simulink model "motor_ctrl_dtc_ver1"  (R2020b)
settings: Solver=VariableStepAuto  StartTime=0.0  StopTime=1  RelTol=1e-3
InitFcn:
  | Rs=0.43;
  | 
  | Lls=0.002
  | 
  | Rr=0.816;
  | 
  | Llr=0.002
  | 
  | Lm=0.6931;
  | 
  | 
  | J=0.085;
  | np=2;
  | 
  | Ts=1e-5;
  | 
  | Udc=400*sqrt(3)
  | Tpwm = 1e-4;
  | 
  | 
  | 
  | Ls = 1.5*Lm+Lls
  | Lr = 1.5*Lm+Llr
  | Tr = Lr/Rr;
  | sigma = (Ls*Lr-Lm*Lm)/Ls/Lr;
model workspace (MAT data in the model file):
  Tsys = 2e-06
  sample_time = 1e-06
libraries: powerlib x17, simulink x3
settings Model: SimulationMode=accelerator  OrderedModelArguments=off  Creator=messer  LastModifiedBy=messer

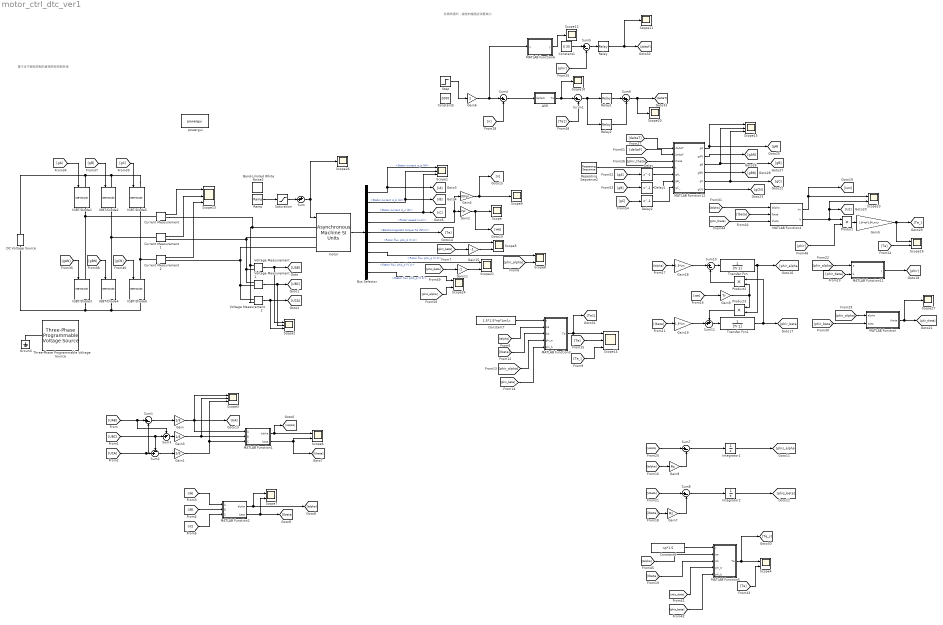
== system motor_ctrl_dtc_ver1 ==
  note: 在高转速时，磁链的幅值应该要减小
  note: 基于定子磁链控制的直接转矩控制系统
  ASR : Subsystem
  Band-Limited White Noise2 : simulink/Sources/Band-Limited White Noise  Cov=[0.0001]  Ts=1e-4  seed=[130341]
  Bus Selector : BusSelector  OutputSignals=Stator measurements.Stator current is_a (A),Stator measurements.Stator current is_b (A),Stator measurements.Stator current is_c (A),Mechanical.Rotor speed (wm),Mechanical.Electromagnetic torque Te (N*m),Rotor measurements.Rotor flux phir_d (V s),Rotor measurements.Rotor flux phir_q (V s),Stator measurements.Stator flux phis_d (V s),Stator measurements.Stator flux phis_q (V s)
  Constant1 : Constant  Value=0.35
  Constant5 : Constant  Value=2000
  Constant6 : Constant  Value=np*1.5
  Constant7 : Constant  Value=1.5*1.5*np*Lm/Lr
  Current Measurement : powerlib/Measurements/Current Measurement  PhasorSimulation=off  OutputType=Complex  PSBequivalent=0
  Current Measurement1 : powerlib/Measurements/Current Measurement  PhasorSimulation=off  OutputType=Complex  PSBequivalent=0
  Current Measurement2 : powerlib/Measurements/Current Measurement  PhasorSimulation=off  OutputType=Complex  PSBequivalent=0
  DC Voltage Source : powerlib/Electrical Sources/DC Voltage Source  Amplitude=Udc  Measurements=None
  Delay : Delay  DelayLength=1  InitialCondition=0
  Delay1 : Delay  DelayLength=1  InitialCondition=0
  Delay2 : Delay  DelayLength=1  InitialCondition=0
  Gain : Gain  Gain=1/3
  Gain1 : Gain  Gain=1/3
  Gain11 : Gain  Gain=-1
  Gain15 : Gain  Gain=-1
  Gain18 : Gain  Gain=1.5*Lm
  Gain19 : Gain  Gain=1.5*Lm
  Gain2 : Gain  Gain=np
  Gain3 : Gain  Gain=1/3
  Gain4 : Gain  Gain=30/pi
  Gain5 : Gain  Gain=1.5*np*1.5*Lm/Lr
  Gain6 : Gain
  Gain7 : Gain  Gain=Rs
  Gain8 : Gain  Gain=Rs
  Gain9 : Gain  Gain=Tr
  Ground : powerlib/Elements/Ground  LConnTagsString=a
  IGBT/Diode{1..6} (6 alike) : powerlib/Power Electronics/IGBT//Diode  Ron=1e-3  Rs=1e5  Cs=inf  Measurements=on
  Integrator1 : Integrator
  Integrator2 : Integrator
  MATLAB Function : MATLAB Function  TreatAsAtomicUnit=on
  MATLAB Function1 : MATLAB Function  TreatAsAtomicUnit=on
  MATLAB Function11 : MATLAB Function  TreatAsAtomicUnit=on
  MATLAB Function12 : MATLAB Function  TreatAsAtomicUnit=on
  MATLAB Function2 : MATLAB Function  TreatAsAtomicUnit=on
  MATLAB Function3 : MATLAB Function  TreatAsAtomicUnit=on
  MATLAB Function4 : MATLAB Function  TreatAsAtomicUnit=on
  MATLAB Function5 : MATLAB Function  TreatAsAtomicUnit=on
  MATLAB Function6 : MATLAB Function  TreatAsAtomicUnit=on
  Product : Product
  Product2 : Product
  Product3 : Product
  Ramp : simulink/Sources/Ramp  slope=100  start=0.25  InitialOutput=5
  Relay : Relay  OnSwitchValue=0.1  OffSwitchValue=-0.1
  Relay1 : Relay  OnSwitchValue=15  OffSwitchValue=10
  Relay2 : Relay  OnSwitchValue=-10  OffSwitchValue=-15  OnOutputValue=0  OffOutputValue=-1
  Repeating Sequence2 : simulink/Sources/Repeating Sequence  rep_seq_t=[0 Tpwm]  rep_seq_y=[0 1]
  Saturation : Saturate  UpperLimit=20  LowerLimit=0
  Scope{,9..12,20,26..27} (8 alike) : Scope
  Scope{1..3,13..15} (6 alike) : Scope  NumInputPorts=3
  Scope{4..8,16,21,23..24} (9 alike) : Scope  NumInputPorts=2
  Step : Step  Time=0.21  Before=2000  After=3000  SampleTime=0
  Su`m1 : Sum  Inputs=|+-
  Sum : Sum  Inputs=++|
  Sum{1,4..5,7..8,10} (6 alike) : Sum  Inputs=|+-
  Sum11 : Sum  Inputs=++|
  Sum2 : Sum  Inputs=-+|
  Sum3 : Sum  Inputs=-+|
  Sum6 : Sum  Inputs=|++
  Three-Phase Programmable Voltage Source : powerlib/Electrical Sources/Three-Phase Programmable Voltage Source  PositiveSequence="[380/sqrt(2)  0 50]"  VariationEntity=None  VariationType=Table of time-amplitude pairs  VariationTypeAlt=Step  VariationStep=0.5  VariationRate=10  VariationMagnitude=0.3  VariationFrequency=2  VariationTiming=[1 2]  VariationPhaseA=off  Amplitudes=[1 0.8 1.2 1.0]  TimeValues=[0 0.1 0.15 0.2]  HarmonicGeneration=off  HarmonicA=[3 0.2 -25 0]  HarmonicB=[2 0.15 35 2]  Timing="[0.05  3]"  BusType=swing  Pref=0  Qref=0  Qmin=-inf  Qmax=inf
  Transfer Fcn : TransferFcn  Denominator=[Tr 1]
  Transfer Fcn1 : TransferFcn  Denominator=[Tr 1]
  Voltage Measurement : powerlib/Measurements/Voltage Measurement  PhasorSimulation=off  OutputType=Complex  PSBequivalent=0
  Voltage Measurement1 : powerlib/Measurements/Voltage Measurement  PhasorSimulation=off  OutputType=Complex  PSBequivalent=0
  Voltage Measurement2 : powerlib/Measurements/Voltage Measurement  PhasorSimulation=off  OutputType=Complex  PSBequivalent=0
  motor : powerlib/Machines/Asynchronous Machine SI Units  RotorType=Squirrel-cage  PresetModel=No  MechanicalLoad=Torque Tm  ShowDetailedParameters=on  ReferenceFrame=Stationary  Units=SI  MeasurementBus=off  NominalParameters=[562000 2750 135]  Stator=[Rs Lls]  Rotor=[Rr Llr]  Cage1=[0.4155 0.002066]  Cage2=[0.4168 0.0003495]  Lm=Lm  Mechanical=[J 0 np]  PolePairs=2  InitialConditions=[1 0 0 0 0 0 0 0]  SimulateSaturation=off  Saturation=[14.03593122, 27.81365428, 53.79336849, 72.68890987, 97.98006896, 148.6815601, 215.7428561, 302.9841135, 428.7778367 ; 230, 322, 414, 460, 506, 552, 598, 644, 690]  LoadFlowParameters=1492000  TsPowergui=0  TsBlock=-1  IterativeModel=Trapezoidal non iterative  IterativeDiscreteModel=Trapezoidal non iterative  Pmec=1.492e+006
  powergui : powerlib/powergui  Priority=1  SimulationMode=Discrete  SampleTime=Tsys  frequency=60  Iterations=50  frequencyindice=0  Pbase=100e6  ErrMax=1e-4  UnitsV=kV  UnitsW=MW  buscounter=0  FunctionMessages=off  echomessages=off  EnableUseOfTLC=off  CurrentSourceSwitches=off  DisableSnubberDevices=off  DisableRonSwitches=off  DisableVfSwitches=off  DisplayEquations=off  AutomaticDiscreteSolvers=off  SolverType=Tustin/Backward Euler (TBE)  Interpol=off  ExternalGateDelay=off  methode=off  Ts=100  x0status=blocks  SPID=on  SwTol=0  HookPort=off  NonlinearTolerance=1e-4  nMaxIteration=100  ContinueOnMaxIteration=off  RestoreLinks=warning  ResistiveCurrentMeasurement=off  Frange=[0:2:500]  Ylog=off  Xlog=on  ShowGrid=off  save=off  variable=ZData  structure=0  ZoomFFT=off  StartTime=0.0  cycles=1  DisplayStyle=1  fundamental=60  FreqAxis=off  MaxFrequency=1000  frequencyindicesteady=1  RmsSteady=1  display=off
  wires:
  Bus Selector/4 -> Gain4/1, Gain2/1  "<Rotor speed (wm)>"
  Bus Selector/2 -> [iB], Scope1/2  "<Stator current is_b (A)>"
  Bus Selector/5 -> [Te]  "<Electromagnetic torque Te (N*m)>"
  Saturation/1 -> Sum/2
  Bus Selector/1 -> [iA], Scope1/1  "<Stator current is_a (A)>"
  motor/1 -> Bus Selector/1
  Bus Selector/3 -> [iC], Scope1/3  "<Stator current is_c (A)>"
  Ramp/1 -> Saturation/1
  Voltage Measurement1/1 -> [UBC], Scope2/2
  Voltage Measurement/1 -> Scope2/1, [UAB]
  Voltage Measurement2/1 -> [UCA], Scope2/3
  [UAB] -> Sum3/1, Sum1/1
  [UCA] -> Sum1/2, Sum2/2
  Sum1/1 -> Gain/1
  [UBC] -> Sum2/1, Sum3/2
  Sum2/1 -> Gain1/1
  Sum3/1 -> Gain3/1
  Gain3/1 -> MATLAB Function1/2(B), Scope3/2
  Gain/1 -> MATLAB Function1/1(A), [UA], Scope3/1
  Gain1/1 -> MATLAB Function1/3(C), Scope3/3
  Sum/1 -> Scope26/1, motor/1
  MATLAB Function1/1(alpha) -> [Ualpha], Scope6/1
  MATLAB Function1/2(beta) -> [Ubeta], Scope6/2
  MATLAB Function2/2(beta) -> [Ibeta], Scope7/2
  [iB] -> MATLAB Function2/2(B)
  MATLAB Function2/1(alpha) -> Scope7/1, [Ialpha]
  [phir_alpha] -> Scope8/2
  [phir_beta] -> Gain15/1
  Gain15/1 -> Scope5/2
  Bus Selector/6 -> Scope5/1  "<Rotor flux phir_d (V s)>"
  Bus Selector/7 -> Scope8/1  "<Rotor flux phir_q (V s)>"
  Gain2/1 -> [we], Scope/1
  [iA] -> MATLAB Function2/1(A)
  [iC] -> MATLAB Function2/3(C)
  Constant7/1 -> MATLAB Function3/1(c)
  [Ialpha] -> MATLAB Function3/2(isa)
  [Ibeta] -> MATLAB Function3/3(isb)
  [phir_alpha] -> MATLAB Function3/4(phi_a)
  [phir_beta] -> MATLAB Function3/5(phi_b)
  MATLAB Function3/1(Te) -> [Te1], Scope14/1
  [Te] -> Scope14/2
  Gain4/1 -> [n], Scope9/1
  Current Measurement1/1 -> Scope13/2
  Current Measurement2/1 -> Scope13/3
  Current Measurement/1 -> Scope13/1
  [Ialpha] -> MATLAB Function4/1(Ialpha)
  [Ibeta] -> MATLAB Function4/2(Ibeta)
  MATLAB Function4/2(It) -> Scope23/2, [Ist], Product/1
  Product/1 -> Gain5/1
  Gain5/1 -> [Te_], Scope16/1
  [Te] -> Scope16/2
  [phir] -> Sum5/2
  Sum5/1 -> Relay/1
  MATLAB Function4/1(Im) -> [Ism], Scope23/1
  [gA] -> IGBT/Diode1/1
  [gAN] -> IGBT/Diode3/1
  [gB] -> IGBT/Diode2/1
  [gBN] -> IGBT/Diode4/1
  [gC] -> IGBT/Diode5/1
  [gCN] -> IGBT/Diode6/1
  [phir_theta] -> MATLAB Function4/3(theta)
  [phir] -> Product/2
  [n] -> Sum4/2
  Relay/1 -> [deltaF], Scope11/1
  Sum4/1 -> ASR/1(deltaN)
  [Te1] -> Su`m1/2
  Su`m1/1 -> Relay2/1, Relay1/1
  Sum10/1 -> Transfer Fcn/1
  Gain18/1 -> Sum10/1
  Sum11/1 -> Transfer Fcn1/1
  Product2/1 -> Sum10/2
  Gain19/1 -> Sum11/2
  [Ibeta] -> Gain19/1
  [Ialpha] -> Gain18/1
  Transfer Fcn/1 -> Product3/2, [phir_alpha]
  [we] -> Gain9/1
  Product3/1 -> Sum11/1
  Gain9/1 -> Product3/1, Product2/2
  Transfer Fcn1/1 -> Product2/1, [phir_beta]
  [phir_alpha] -> MATLAB Function11/1(a)
  [phir_beta] -> MATLAB Function11/2(b)
  [phir_beta] -> MATLAB Function/2(beta)
  [phir_alpha] -> MATLAB Function/1(alpha)
  MATLAB Function11/1(y) -> [phir]
  MATLAB Function/1(theta) -> Scope27/1, [phir_theta]
  [Te_] -> Scope14/3
  ASR/1(Te) -> Su`m1/1, Scope10/1
  [phis_alpha] -> MATLAB Function5/4(phi_a)
  [Ialpha] -> MATLAB Function5/2(isa)
  [Ialpha] -> Gain8/1
  [Ibeta] -> MATLAB Function5/3(isb)
  Gain7/1 -> Sum8/2
  Integrator2/1 -> [phis_beta]
  Integrator1/1 -> [phis_alpha]
  [Te] -> Scope4/2
  [phis_beta] -> MATLAB Function5/5(phi_b)
  [Ubeta] -> Sum8/1
  Gain8/1 -> Sum7/2
  [Ibeta] -> Gain7/1
  Constant6/1 -> MATLAB Function5/1(c)
  Sum7/1 -> Integrator1/1
  MATLAB Function5/1(Te) -> Scope4/1, [Te_s]
  Sum8/1 -> Integrator2/1
  [Ualpha] -> Sum7/1
  Gain11/1 -> Scope21/2
  [phis_beta] -> Gain11/1
  Bus Selector/8 -> Scope21/1  "<Stator flux phis_d (V s)>"
  [phis_alpha] -> Scope24/2
  Bus Selector/9 -> Scope24/1  "<Stator flux phis_q (V s)>"
  Relay1/1 -> Sum6/1
  Relay2/1 -> Sum6/2
  Repeating Sequence2/1 -> MATLAB Function12/4(t)
  [phir_theta] -> MATLAB Function12/3(theta)
  Sum6/1 -> Scope20/1, [deltaT]
  [deltaT] -> MATLAB Function12/1(deltaT)
  [deltaF] -> MATLAB Function12/2(deltaF)
  MATLAB Function12/2(gAN) -> [gAN]
  MATLAB Function12/6(gCN) -> [gCN]
  MATLAB Function12/5(gC) -> Scope15/3, [gC]
  MATLAB Function12/3(gB) -> Scope15/2, [gB]
  MATLAB Function12/4(gBN) -> [gBN]
  MATLAB Function12/1(gA) -> Scope15/1, [gA]
  Delay/1 -> MATLAB Function12/5(gA_)
  [gA] -> Delay/1
  [gB] -> Delay1/1
  [gC] -> Delay2/1
  Delay1/1 -> MATLAB Function12/6(gB_)
  Delay2/1 -> MATLAB Function12/7(gC_)
  MATLAB Function6/1(y) -> Scope12/1
  Constant1/1 -> Sum5/1
  Gain6/1 -> MATLAB Function6/1(u), Sum4/1
  Step/1 -> Gain6/1
  connections:
  Voltage Measurement1/LConn1 -- Voltage Measurement/LConn2 -- motor/LConn2 -- Current Measurement1/RConn1
  Voltage Measurement2/LConn1 -- Voltage Measurement1/LConn2 -- Current Measurement2/RConn1 -- motor/LConn3
  Voltage Measurement/LConn1 -- Voltage Measurement2/LConn2 -- Current Measurement/RConn1 -- motor/LConn1
  Ground/LConn1 -- Three-Phase Programmable Voltage Source/LConn1
  IGBT/Diode2/RConn1 -- IGBT/Diode4/LConn1 -- Current Measurement1/LConn1
  IGBT/Diode5/LConn1 -- DC Voltage Source/RConn1 -- IGBT/Diode1/LConn1 -- IGBT/Diode2/LConn1
  IGBT/Diode5/RConn1 -- IGBT/Diode6/LConn1 -- Current Measurement2/LConn1
  IGBT/Diode3/RConn1 -- DC Voltage Source/LConn1 -- IGBT/Diode4/RConn1 -- IGBT/Diode6/RConn1
  IGBT/Diode1/RConn1 -- IGBT/Diode3/LConn1 -- Current Measurement/LConn1

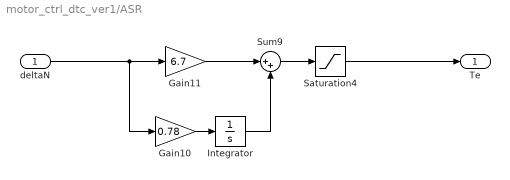
== system motor_ctrl_dtc_ver1/ASR ==
  deltaN : Inport
  Gain10 : Gain  Gain=0.78
  Gain11 : Gain  Gain=6.7
  Integrator : Integrator
  Saturation4 : Saturate  UpperLimit=300  LowerLimit=-300
  Sum9 : Sum  Inputs=|++
  Te : Outport
  wires:
  Gain11/1 -> Sum9/1
  deltaN/1 -> Gain11/1, Gain10/1
  Saturation4/1 -> Te/1
  Gain10/1 -> Integrator/1
  Sum9/1 -> Saturation4/1
  Integrator/1 -> Sum9/2

== matlab function motor_ctrl_dtc_ver1/MATLAB Function1 ==
  data: A input; alpha output; B input; C input; beta output
function [alpha, beta] = fcn(A, B, C)
k = 2/ 3;
alpha = k * (A - 0.5*B - 0.5*C);
beta = k * sqrt(3) / 2 * (B - C);

== matlab function motor_ctrl_dtc_ver1/MATLAB Function5 ==
  data: c input; Te output; isa input; isb input; phi_a input; phi_b input
function Te = fcn(c, isa, isb, phi_a, phi_b)
Te = c *( isb * phi_a - isa * phi_b);

== matlab function motor_ctrl_dtc_ver1/MATLAB Function2 ==
  data: A input; alpha output; B input; C input; beta output
function [alpha, beta] = fcn(A, B, C)
k = 2/ 3;
alpha = k * (A - 0.5*B - 0.5*C);
beta = k * sqrt(3) / 2 * (B - C);

== matlab function motor_ctrl_dtc_ver1/MATLAB Function3 ==
  data: c input; Te output; isa input; isb input; phi_a input; phi_b input
function Te = fcn(c, isa, isb, phi_a, phi_b)
Te = c *( isb * phi_a - isa * phi_b);

== matlab function motor_ctrl_dtc_ver1/MATLAB Function4 ==
  data: Im output; Ialpha input; Ibeta input; theta input; It output
function [Im, It] = fcn(Ialpha, Ibeta, theta)

Im = Ialpha * cos(theta) + Ibeta * sin(theta);
It = -Ialpha * sin(theta) + Ibeta * cos(theta);

== matlab function motor_ctrl_dtc_ver1/MATLAB Function11 ==
  data: y output; a input; b input
function y = fcn(a, b)

y = sqrt(a*a + b*b);

== matlab function motor_ctrl_dtc_ver1/MATLAB Function6 ==
  data: u input; y output
function y = fcn(u)
F = 1.1;
V = 1200;
if(abs(u) <= V )
    y = F;
else
    y = F*V/abs(u);
end

== matlab function motor_ctrl_dtc_ver1/MATLAB Function ==
  data: theta output; alpha input; beta input
function theta = fcn(alpha, beta)

if(beta >=0)
    if(alpha == 0)
        theta = pi/2;
    elseif(alpha >0)
        theta = atan(beta/alpha);
    else
        theta = pi + atan(beta/alpha);
    end
else
    if(alpha == 0)
        theta = 1.5*pi;
    elseif(alpha > 0)
        theta = 2*pi + atan(beta/alpha);
    else
        theta = pi + atan(beta/alpha);
    end
end

== matlab function motor_ctrl_dtc_ver1/MATLAB Function12 ==
  data: gA output; deltaT input; deltaF input; theta input; t input; gAN output; gB output; gBN output; gC output; gCN output; gA_ input; gB_ input; gC_ input
function [gA, gAN, gB, gBN, gC, gCN] = fcn(deltaT, deltaF, theta, t, gA_, gB_, gC_)

% ABC 三个桥的开关
ABC = [gA_, gB_, gC_];

% 六个电压矢量对应的上桥臂开关情况
u0 = [0, 0, 0];
u1 = [1, 0, 0];
u2 = [1, 1, 0];
u3 = [0, 1, 0];
u4 = [0, 1, 1];
u5 = [0, 0, 1];
u6 = [1, 0, 1];
u7 = [1, 1, 1];

% 每个扇区的大小，为 60°
seg = pi / 3;

deltaT = deltaT + 1; % 把 deltaT 从 -1， 0， 1 映射到 0， 1， 2
% 注意，直接转矩扇区和电压矢量扇区是有30度的差距，
theta = mod(theta, 2*pi) + pi / 6; 
sec = int32(theta / seg);
sec = mod(sec, 6);

% deltaIdx 是为了表示方便，用 deltaT 和 deltaF 来进行表示
% 0~2 表示 deltaF = 0下的三个转矩变换调整量
% 3~5 表示 deltaF = 1下的三个转矩变换调整量
deltaIdx = deltaF * 3 + deltaT;

% 在固定周期进行开关管参数更新
if(t >= 0.95) 
    if(sec == 0) % 第一个扇区
        if(deltaIdx == 0) % deltaF = 0, deltaT = -1
            ABC = u5;
        elseif(deltaIdx == 1) 
            ABC = u0;
        elseif(deltaIdx == 2)
            ABC = u3;
        elseif(deltaIdx == 3)
            ABC = u6;
        elseif(deltaIdx == 4)
            ABC = u7;
        else
            ABC = u2;
        end
    elseif(sec == 1) % 第二个扇区
        if(deltaIdx == 0) 
            ABC = u6;
        elseif(deltaIdx == 1) 
            ABC = u7;
        elseif(deltaIdx == 2)
            ABC = u4;
        elseif(deltaIdx == 3)
            ABC = u1;
        elseif(deltaIdx == 4)
            ABC = u0;
        else
            ABC = u3;
        end
    elseif(sec == 2) % 第三个扇区
        if(deltaIdx == 0) 
            ABC = u1;
        elseif(deltaIdx == 1) 
            ABC = u0;
        elseif(deltaIdx == 2)
            ABC = u5;
        elseif(deltaIdx == 3)
            ABC = u2;
        elseif(deltaIdx == 4)
            ABC = u7;
        else
            ABC = u4;
        end
    elseif(sec == 3) % 第四个扇区
        if(deltaIdx == 0) 
            ABC = u2;
        elseif(deltaIdx == 1) 
            ABC = u7;
        elseif(deltaIdx == 2)
            ABC = u6;
        elseif(deltaIdx == 3)
            ABC = u3;
        elseif(deltaIdx == 4)
            ABC = u0;
        else
            ABC = u5;
        end
    elseif(sec == 4) % 第五个扇区
        if(deltaIdx == 0) 
            ABC = u3;
        elseif(deltaIdx == 1) 
            ABC = u0;
        elseif(deltaIdx == 2)
            ABC = u1;
        elseif(deltaIdx == 3)
            ABC = u4;
        elseif(deltaIdx == 4)
            ABC = u7;
        else
            ABC = u6;
        end
    else % 最后一个扇区，第6扇区
        if(deltaIdx == 0) 
            ABC = u4;
        elseif(deltaIdx == 1) 
            ABC = u7;
        elseif(deltaIdx == 2)
            ABC = u2;
        elseif(deltaIdx == 3)
            ABC = u5;
        elseif(deltaIdx == 4)
            ABC = u0;
        else
            ABC = u1;
        end
    end
end

gA = ABC(1);
gAN = ~gA;
gB = ABC(2);
gBN = ~gB;
gC = ABC(3);
gCN = ~gC;
% g = [gA, ~gA, gB, ~gB, gC, ~gC];
